simulink model "PIDimpedencecontrol"  (R2018b)
settings: Solver=ode1  StartTime=0.0  StopTime=inf  FixedStep=0.01  RelTol=1e-3
undefined symbols (not defined in the file or in its folder): ai0, Dev1
libraries: simulink x3, NIDAQ_Library x1
settings Model: Creator=Spider PC  LastModifiedBy=Spider PC
settings SolverCC: AlgebraicLoopSolver=LineSearch
settings SFSimCC: SimUseLocalCustomCode=off
settings RTWCC: RTWUseLocalCustomCode=off

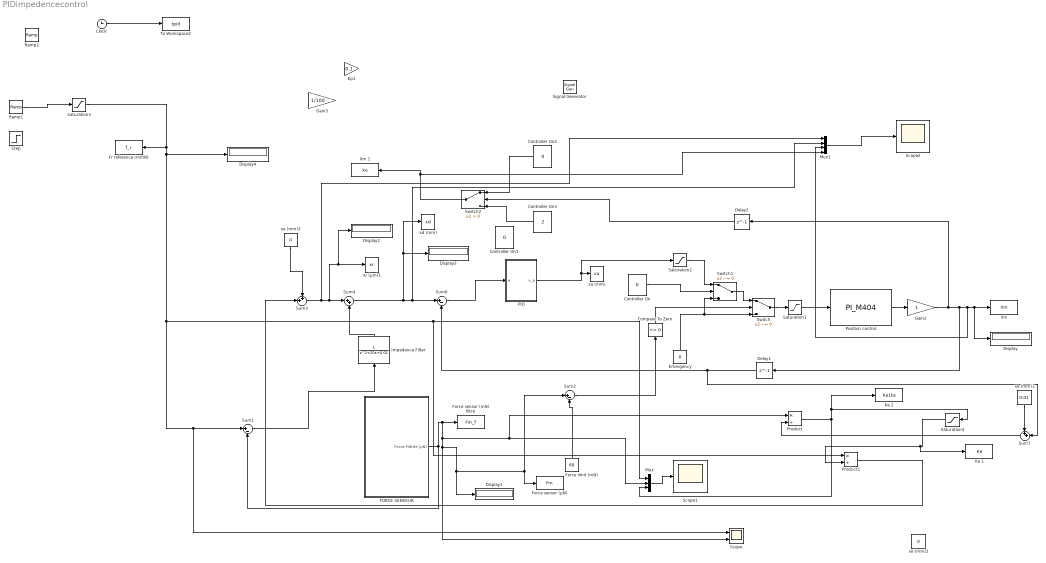
== system PIDimpedencecontrol ==
  Clock : Clock
  Compare To Zero : simulink/Logic and Bit Operations/Compare To Zero  relop=<=  OutDataTypeStr=uint8
  Controller On : Constant  Value=0
  Controller On1 : Constant  Value=0
  Controller On2 : Constant  Value=0
  Controller On3 : Constant  Value=2
  Delay1 : Delay  DelayLength=1  InitialCondition=0
  Delay2 : Delay  DelayLength=1  InitialCondition=0
  Display{,1..4} (5 alike) : Display
  Emergency : Constant  Value=0
  FORCE SENSEUR : Subsystem
  Force limit (mN) : Constant  Value=60
  Force sensor (mN) filtré : ToWorkspace  VariableName=Fm_f  SampleTime=-1
  Force sensor (µN) : ToWorkspace  VariableName=Fm  SampleTime=-1
  Fr reference (mmN) : ToWorkspace  VariableName=f_r  SampleTime=-1
  Gain2 : Gain
  Gain3 : Gain  Gain=1/100
  Impedance Filter : TransferFcn  Numerator=1  Denominator=[1 20 0.01]
  Ke 1 : ToWorkspace  VariableName=Ke  SampleTime=-1
  Ke 2 : ToWorkspace  VariableName=Ke1bs  SampleTime=-1
  Kp1 : Gain  Gain=0.1
  Mux : Mux  Inputs=3
  Mux1 : Mux
  PID : Subsystem
  Position control : S-Function  FunctionName=PI_M404  SFunctionDeploymentMode=off  EnableBusSupport=off
  Product : Product  Inputs=*/
  Product1 : Product  Inputs=*/
  Ramp1 : simulink/Sources/Ramp  slope=0.1  start=10  InitialOutput=0
  Ramp2 : simulink/Sources/Ramp  slope=0.1  start=0  InitialOutput=0
  Saturation1 : Saturate  UpperLimit=70  LowerLimit=0
  Saturation2 : Saturate  UpperLimit=20  LowerLimit=0
  Saturation3 : Saturate  UpperLimit=10  LowerLimit=0
  Saturation4 : Saturate  UpperLimit=300  LowerLimit=0.01
  Scope : Scope  NumInputPorts=2
  Scope1 : Scope
  Scope2 : Scope
  Signal Generator : SignalGenerator  Units=rad/sec
  Step : Step  Time=3  After=2
  Sum1 : Sum  Inputs=|+-
  Sum2 : Sum  Inputs=|+-
  Sum3 : Sum  Inputs=++|
  Sum4 : Sum  Inputs=|++
  Sum6 : Sum  Inputs=|+-
  Sum7 : Sum  Inputs=++|
  Switch : Switch  Criteria=u2 ~= 0
  Switch1 : Switch  Criteria=u2 ~= 0
  Switch2 : Switch  Criteria=u2 > Threshold
  To Workspace2 : ToWorkspace  VariableName=tpid  SampleTime=-1
  "Xm " : ToWorkspace  VariableName=Xm  SampleTime=-1
  Xm 1 : ToWorkspace  VariableName=Xe  SampleTime=-1
  xa (mm) : ToWorkspace  VariableName=xa  SampleTime=-1
  xd (mm) : ToWorkspace  VariableName=xd  SampleTime=-1
  xe (mm)1 : Constant  Value=0.01
  xe (mm)2 : Constant  Value=0
  xe (mm)3 : Constant  Value=0
  xr (µm)1 : ToWorkspace  VariableName=xr  SampleTime=-1
  wires:
  Clock/1 -> To Workspace2/1
  PID/1(x_a) -> Saturation2/1, xa (mm)/1
  Switch1/1 -> Switch/1
  Force limit (mN)/1 -> Sum2/2
  Emergency/1 -> Switch/3, Switch1/3
  Sum2/1 -> Compare To Zero/1
  Switch/1 -> Saturation1/1
  Compare To Zero/1 -> Switch/2
  Position control/1 -> Gain2/1
  Saturation1/1 -> Position control/1
  FORCE SENSEUR/1(Force Filtrée (µN)) -> Product/1, Mux/2, Display1/1, Force sensor (µN)/1, Sum2/1, Scope/2, Force sensor (mN) filtré/1, Sum1/2
  Sum1/1 -> Impedance Filter/1
  Impedance Filter/1 -> Sum4/2
  Sum3/1 -> Mux1/1, Display2/1, xr (µm)1/1, Sum4/1
  Sum6/1 -> PID/1(e)
  Gain2/1 -> Delay2/1, Delay1/1, Mux1/3, "Xm "/1, Display/1
  Delay1/1 -> Sum7/2, Sum6/2
  xe (mm)1/1 -> Sum7/1
  Controller On/1 -> Switch1/2
  Saturation3/1 -> Display4/1, Product1/1, Mux/1, Scope/1, Sum1/1, Fr reference (mmN)/1
  Switch2/1 -> Mux1/4, Xm 1/1
  Controller On2/1 -> Switch2/1
  Controller On3/1 -> Switch2/3
  Mux/1 -> Scope1/1
  Mux1/1 -> Scope2/1
  Delay2/1 -> Switch2/2
  Product/1 -> Saturation4/1, Ke 2/1, Mux/3
  Product1/1 -> Sum3/2
  Sum4/1 -> Mux1/2, Sum6/1, Display3/1, xd (mm)/1
  Saturation4/1 -> Ke 1/1, Product1/2
  Saturation2/1 -> Switch1/1
  Sum7/1 -> Product/2
  xe (mm)3/1 -> Sum3/1
  Ramp1/1 -> Saturation3/1

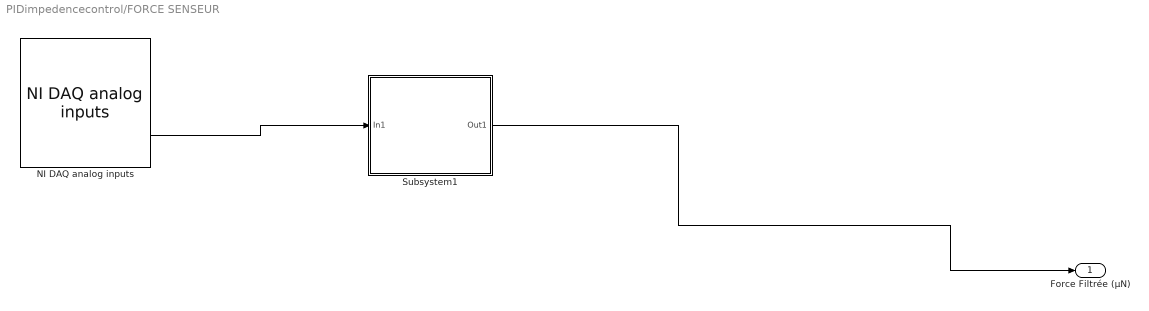
== system PIDimpedencecontrol/FORCE SENSEUR ==
  NI DAQ analog inputs : NIDAQ_Library/NI DAQ analog inputs  NBCHAN=1  CHANNELS=Dev1/ai0  STEP=0.01  MINVAL=-10  MAXVAL=10  TERMCFG=DAQmx_Val_Diff
      settings: SourceProductName=NI-DAQ
  Subsystem1 : Subsystem
  Force Filtrée (µN) : Outport
  wires:
  NI DAQ analog inputs/2 -> Subsystem1/1(In1)
  Subsystem1/1(Out1) -> Force Filtrée (µN)/1

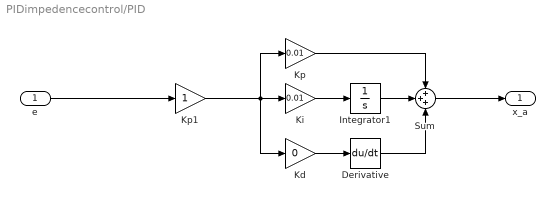
== system PIDimpedencecontrol/PID ==
  e : Inport
  Derivative : Derivative
  Integrator1 : Integrator
  Kd : Gain  Gain=0
  Ki : Gain  Gain=0.01
  Kp : Gain  Gain=0.01
  Kp1 : Gain
  Sum : Sum  Inputs=+++
  x_a : Outport
  wires:
  Derivative/1 -> Sum/3
  Integrator1/1 -> Sum/2
  Kp/1 -> Sum/1
  e/1 -> Kp1/1
  Ki/1 -> Integrator1/1
  Kd/1 -> Derivative/1
  Sum/1 -> x_a/1
  Kp1/1 -> Kp/1, Ki/1, Kd/1

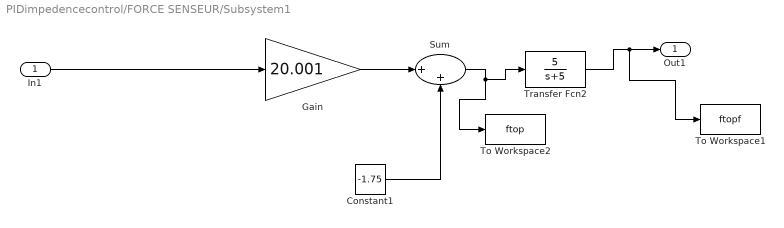
== system PIDimpedencecontrol/FORCE SENSEUR/Subsystem1 ==
  In1 : Inport
  Constant1 : Constant  Value=-1.75
  Gain : Gain  Gain=20.001
  Sum : Sum  Inputs=|++
  To Workspace1 : ToWorkspace  VariableName=ftopf  SampleTime=-1
  To Workspace2 : ToWorkspace  VariableName=ftop  SampleTime=-1
  Transfer Fcn2 : TransferFcn  Numerator=[5]  Denominator=[1 5]
  Out1 : Outport
  wires:
  Constant1/1 -> Sum/2
  Gain/1 -> Sum/1
  Sum/1 -> Transfer Fcn2/1, To Workspace2/1
  In1/1 -> Gain/1
  Transfer Fcn2/1 -> To Workspace1/1, Out1/1
